simulink subsystem "CF2_SubSystem"  (R2020b)
settings: Solver=VariableStepAuto  StartTime=0.0  StopTime=10.0  RelTol=1e-3
values from neighbouring files (symbols this model uses):
  C = Ts/(Ts + Tc)    [StateSpaceSimpleObserver.m]
undefined symbols (not defined in the file or in its folder): Ts
settings Model: Creator=umberto  LastModifiedBy=umberto

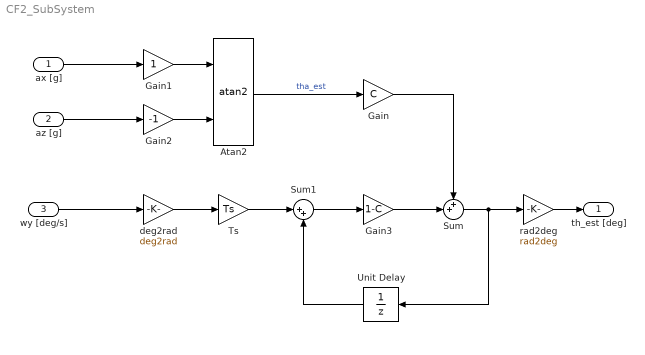
== system CF2_SubSystem ==
  ax [g] : Inport
  az [g] : Inport  Port=2
  wy [deg/s] : Inport  Port=3
  Atan2 : Trigonometry  Operator=atan2
  Gain : Gain  Gain=C
  Gain1 : Gain
  Gain2 : Gain  Gain=-1
  Gain3 : Gain  Gain=1-C
  Sum : Sum  Inputs=++|
  Sum1 : Sum  Inputs=|++
  Ts : Gain  Gain=Ts
  Unit Delay : UnitDelay  SampleTime=-1  HasFrameUpgradeWarning=on
  deg2rad : Gain  Gain=deg2rad
  rad2deg : Gain  Gain=rad2deg
  th_est [deg] : Outport
  wires:
  wy [deg/s]/1 -> deg2rad/1
  deg2rad/1 -> Ts/1
  ax [g]/1 -> Gain1/1
  az [g]/1 -> Gain2/1
  Gain1/1 -> Atan2/1
  Gain2/1 -> Atan2/2
  Atan2/1 -> Gain/1  "tha_est"
  Sum/1 -> Unit Delay/1, rad2deg/1
  rad2deg/1 -> th_est [deg]/1
  Gain/1 -> Sum/1
  Ts/1 -> Sum1/1
  Gain3/1 -> Sum/2
  Sum1/1 -> Gain3/1
  Unit Delay/1 -> Sum1/2
